simulink model "PMSM_SVC_RHF"  (R2019b)
settings: Solver=ode1  StartTime=0.0  StopTime=10  FixedStep=Tsim  RelTol=1e-3  EnableMultiTasking=on
PostLoadFcn:
  | , if any(exist('dsrtsu_mdlpostloadfcn', 'file') == [2, 3, 6]), try dsrtsu_mdlpostloadfcn('Execute', bdroot); catch fprintf('Error in PostLoadFcn (dsrtsu_mdlpostloadfcn) for model "%s":\n %s\n', bdroot, lasterr); end, end,
undefined symbols (not defined in the file or in its folder): bw_BPF, DiscIntNeverNeededParam, f_HF, Flux, fpwm, Fr, i_max, Jm, Ld, Lq, Ls, p, Rs, T_max, Tcur, Tsim, u_max, Udc, v_HF
libraries: powerlib x4, powerlib_meascontrol x4, simulink x1, powerlib_extras x1
settings Model: DSRTSU_INTERNAL_RTI_VER=490  DSRTSU_INTERNAL_RTI_TYPE=rti1202  SimulationMode=accelerator  Creator=XIL1XI  LastModifiedBy=LEI
settings SolverCC: AutoInsertRateTranBlk=on
settings DataIOCC: LimitDataPoints=on  ReturnWorkspaceOutputs=off
settings OptimizationCC: BlockReduction=off  OptimizeBlockIOStorage=off  BufferReuse=off  GlobalBufferReuse=off  ExpressionFolding=off  LocalBlockOutputs=off  LifeSpan=inf  OptimizeDataStoreBuffers=off  BusAssignmentInplaceUpdate=off
settings DebuggingCC: AllowSymbolicDim=off  SFUnexpectedBacktrackingDiag=warning  SFNoUnconditionalDefaultTransitionDiag=warning  SFExecutionAtInitializationDiag=none  ArithmeticOperatorsInVariantConditions=warning
settings HardwareCC: ProdBitPerPointer=32  ProdBitPerSizeT=32  ProdBitPerPtrDiffT=32  ProdLargestAtomicInteger=Integer  ProdEndianess=BigEndian  ProdWordSize=32  ProdHWDeviceType=Custom Processor->Custom
settings ModelReferenceCC: PropagateSignalLabelsOutOfModel=off
settings SFSimCC: SimUseLocalCustomCode=off  CustomCodeUndefinedFunction=UseInterfaceOnly
settings RTWCC: Description=dSPACE DS1202 Hardware Platform  SystemTargetFile=rti1202.tlc  MakeCommand=make_rti  TemplateMakefile=rti1202.tmf  RTWUseLocalCustomCode=off
settings CodeAppCC: StateflowObjectComments=on
settings STFCustomTargetCC: ModelReferenceCompliant=off  ParMdlRefBuildCompliant=on  MatFileLogging=on  SystemTargetFile=rti1202.tlc
settings GRTTargetCC: TargetLangStandard=C89/C90 (ANSI)  ModelReferenceCompliant=off  CompOptLevelCompliant=off  ConcurrentExecutionCompliant=off  CombineOutputUpdateFcns=off  CPPClassGenCompliant=off  UseToolchainInfoCompliant=off
settings ConfigComp: CovMetricSettings=dw  CovHtmlReporting=on  CovSaveCumulativeToWorkspaceVar=on  CovSaveSingleToWorkspaceVar=on  CovExternalEMLEnable=off
settings SimscapeCC: SimscapeNormalizeSystem=off

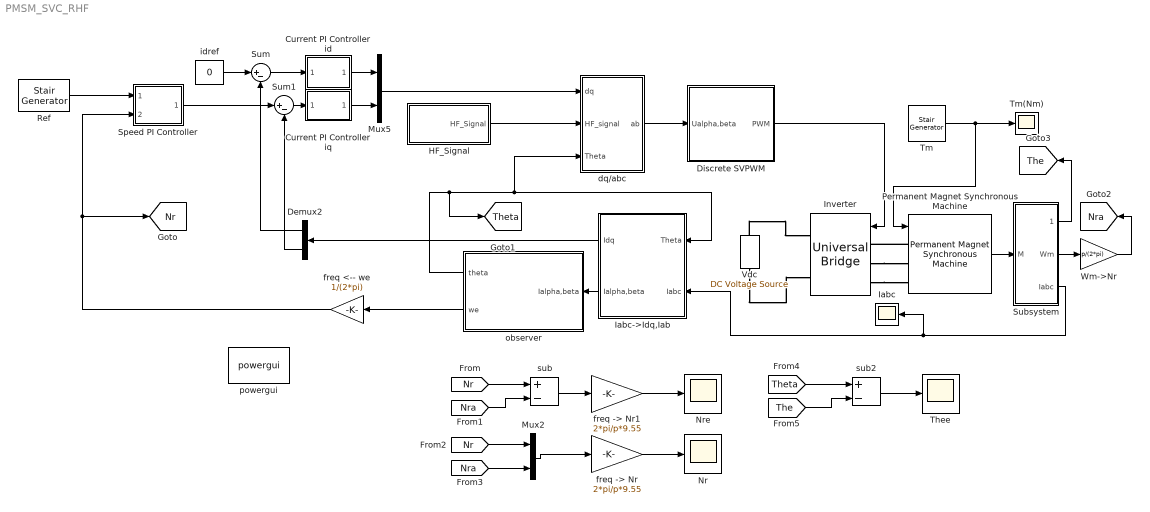
== system PMSM_SVC_RHF ==
  " Current PI Controller iq" : Subsystem  mask(Current PI Controller){Rs=Rs, Ls=Ld, fpwm=fpwm, Par_Limits=[u_max -u_max], T=Tcur, kp_gain=1, ti_gain=1}
      mask prompts: Rs "Stator resistance Rs (ohm):"; Ls "Stator inductance Ls (H):"; fpwm "PWM frequency fpwm (Hz):"; Par_Limits "Output limits Par_Limits (V): [ Upper   Lower ]"; T "Sample time T (s):"
      mask help:
      | Kp, Ti can be calculated automatically:
      |
      |     kp = Ls/2*fpwm;
      |     ti = Ls/Rs;
      |     ki = kp/ti;
      |
      | Kp_Gain, Ki_Gain are used to adjust the calculated kp and ki. Controller limit is the integrator saturation limit and the output limit.
      mask Display: disp('PI');
  Current PI Controller id : Subsystem  mask(Current PI Controller){Rs=Rs, Ls=Ld, fpwm=fpwm, Par_Limits=[u_max -u_max], T=Tcur, kp_gain=1, ti_gain=1}
      mask prompts: Rs "Stator resistance Rs (ohm):"; Ls "Stator inductance Ls (H):"; fpwm "PWM frequency fpwm (Hz):"; Par_Limits "Output limits Par_Limits (V): [ Upper   Lower ]"; T "Sample time T (s):"
      mask help:
      | Kp, Ti can be calculated automatically:
      |
      |     kp = Ls/2*fpwm;
      |     ti = Ls/Rs;
      |     ki = kp/ti;
      |
      | Kp_Gain, Ki_Gain are used to adjust the calculated kp and ki. Controller limit is the integrator saturation limit and the output limit.
      mask Display: disp('PI');
  Demux2 : Demux  Outputs=2
  Discrete SVPWM : Subsystem  mask(Seven - sects SVPWM generator){td=0, fpwm=fpwm, T=Tsim}
      mask prompts: td "Dead Time td (s):"; fpwm "PWM frequency fpwm (Hz):"; T "Sample time T (s):"
      mask help: This block implements a space vector PWM.
  HF_Signal : Subsystem
  Iabc : Scope
  Iabc->Idq,Iab : Subsystem  mask(Transformation abc to ab and dq){T=Tcur}
      mask prompts: T "Sample time T (s):"
  Inverter : powerlib/Power Electronics/Universal Bridge  Arms=3  SnubberResistance=1e5  SnubberCapacitance=inf  Device=IGBT / Diodes  Ron=1e-3  Lon=0  ForwardVoltages=[0,0]  ForwardVoltage=0  GTOparameters=[ 10e-6 , 20e-6 ]  IGBTparameters=[0,0]  Measurements=None  Measurements_2=None  converterType=Rectifier
      settings: SourceProductName=Simscape Electrical
  Mux2 : Mux  Inputs=2
  Mux5 : Mux  Inputs=2
  Nr : Scope
  Nre : Scope
  Permanent Magnet Synchronous Machine : powerlib/Machines/Permanent Magnet Synchronous Machine  NbPhases=3  FluxDistribution=Sinusoidal  RotorType=Salient-pole  MechanicalLoad=Torque Tm  PresetModel=No  ShowDetailedParameters=on  MeasurementBus=off  Resistance=Rs  Inductance=8.5e-3  dqInductances=[Ld,Lq]  La=Ls  MachineConstant=Flux linkage established by magnets (V.s)  Flux=Flux  VoltageCst=161.7909  TorqueCst=1.338  Flat=120  Mechanical=[Jm Fr p 0]  PolePairs=4  InitialConditions=[0,0, 0,0]  InitialConditions5ph=[0 0 0 0 0 0]  RefAngle=Aligned with phase A axis (original Park)  IterativeDiscreteModel=Trapezoidal non iterative  TsBlock=-1  TsPowergui=0
  Ref : powerlib_meascontrol/Pulse & Signal Generators/Stair Generator  t="[0  2  6 ]"  e=[0 10 20]  Ts=Tcur
      settings: SourceProductName=Simscape Electrical
  Speed PI Controller : Subsystem  mask(Speed PI Controller){kp=2.5, ti=2.5/10, Par_Limits=[T_max -T_max], T=Tcur}
      mask prompts: kp "proportional gain"; ti "integral time"; Par_Limits "Output limits: [ Upper   Lower ]"; T "Sample time T (s):"
      mask help:
      | Kp, Ti can be calculated automatically:
      |
      |     kp = Jm*(h+1)/(2*h*2*fpwm*kt)*kp_gain;
      |     ki = Jm*(h+1)/(2*h*2*fpwm*kt)/(2*1/fpwm)*ti_gain;
      |     ti = kp/ki;
      |
      |
      | Kp_Gain, Ki_Gain are used to adjust the calculated kp and ki. Controller limit is the integrator saturation limit and the output limit.
      mask init:
      | UpperLimit=Par_Limits(1);
      | LowerLimit=Par_Limits(2);
      | 
      | ki = kp/ti;
      mask Display: disp('PI')
  Subsystem : Subsystem
  Sum : Sum  Inputs=|+-
  Sum1 : Sum  Inputs=|+-
  Thee : Scope
  Tm : powerlib_meascontrol/Pulse & Signal Generators/Stair Generator  t="[0  4 ]"  e=[0 3 ]  Ts=0
      settings: SourceProductName=Simscape Electrical
  Tm(Nm) : Scope
  Vdc : powerlib/Electrical Sources/DC Voltage Source  Amplitude=Udc  Measurements=None
      settings: SourceProductName=Simscape Electrical
  Wm->Nr : Gain  Gain=p/(2*pi)
  dq/abc : Subsystem
  "freq -> Nr" : Gain  Gain=2*pi/p*9.55
  "freq -> Nr1" : Gain  Gain=2*pi/p*9.55
  freq <-- we : Gain  Gain=1/(2*pi)
  idref : Constant  Value=0
  observer : Subsystem
  powergui : powerlib/powergui  Priority=1  SimulationMode=Discrete  SampleTime=Tsim  frequency=60  Iterations=50  frequencyindice=0  Pbase=100e6  ErrMax=1e-4  UnitsV=kV  UnitsW=MW  buscounter=0  FunctionMessages=off  echomessages=off  EnableUseOfTLC=off  CurrentSourceSwitches=off  DisableSnubberDevices=off  DisableRonSwitches=off  DisableVfSwitches=off  DisplayEquations=off  AutomaticDiscreteSolvers=off  SolverType=Tustin/Backward Euler (TBE)  Interpol=off  ExternalGateDelay=off  methode=off  Ts=10  x0status=blocks  SPID=off  SwTol=0  HookPort=off  NonlinearTolerance=1e-4  nMaxIteration=100  ContinueOnMaxIteration=off  RestoreLinks=warning  ResistiveCurrentMeasurement=off  Frange=[0:2:500]  Ylog=off  Xlog=on  ShowGrid=off  save=off  variable=ZData  structure=0  ZoomFFT=off  StartTime=0.0  cycles=1  DisplayStyle=1  fundamental=60  FreqAxis=off  MaxFrequency=1000  frequencyindicesteady=1  RmsSteady=1  display=off
      settings: SourceProductName=Simscape Electrical
  sub : Sum  Inputs=+-
  sub2 : Sum  Inputs=+-
  tag scope: Nr=global, Nra=global, The=global, Theta=global
  wires:
  Current PI Controller id/1(U_Ref) -> Mux5/1
  " Current PI Controller iq"/1(U_Ref) -> Mux5/2
  observer/2(we) -> freq <-- we/1
  Mux2/1 -> "freq -> Nr"/1
  Mux5/1 -> dq/abc/1(dq)
  dq/abc/1(ab) -> Discrete SVPWM/1(Ualpha,beta)
  Iabc->Idq,Iab/1(Idq) -> Demux2/1
  Iabc->Idq,Iab/2(Ialpha,beta) -> observer/1(Ialpha,beta)
  Tm/1 -> Permanent Magnet Synchronous Machine/1, Tm(Nm)/1
  sub/1 -> "freq -> Nr1"/1
  Ref/1 -> Speed PI Controller/1(f_ref)
  Permanent Magnet Synchronous Machine/1 -> Subsystem/1(M)
  HF_Signal/1(HF_Signal) -> dq/abc/2(HF_signal)
  Discrete SVPWM/1(PWM) -> Inverter/1
  Subsystem/3(Iabc) -> Iabc/1, Iabc->Idq,Iab/2(Iabc)
  "freq -> Nr"/1 -> Nr/1
  "freq -> Nr1"/1 -> Nre/1
  Demux2/1 -> Sum/2
  Subsystem/2(Wm) -> Wm->Nr/1
  observer/1(theta) -> [Theta], Iabc->Idq,Iab/1(Theta), dq/abc/3(Theta)
  freq <-- we/1 -> [Nr], Speed PI Controller/2(f_fed)
  [Nr] -> sub/1
  Wm->Nr/1 -> [Nra]
  [Nra] -> sub/2
  [Nr] -> Mux2/1
  [Nra] -> Mux2/2
  Subsystem/1(Them) -> [The]
  [Theta] -> sub2/1
  [The] -> sub2/2
  sub2/1 -> Thee/1
  Sum/1 -> Current PI Controller id/1(I_Ref)
  Sum1/1 -> " Current PI Controller iq"/1(I_Ref)
  Speed PI Controller/1(Te_Ref) -> Sum1/1
  Demux2/2 -> Sum1/2
  idref/1 -> Sum/1
  connections:
  Inverter/LConn2 -- Permanent Magnet Synchronous Machine/LConn2
  Permanent Magnet Synchronous Machine/LConn1 -- Inverter/LConn1
  Inverter/LConn3 -- Permanent Magnet Synchronous Machine/LConn3
  Vdc/RConn1 -- Inverter/RConn1
  Vdc/LConn1 -- Inverter/RConn2

== system PMSM_SVC_RHF/ Current PI Controller iq ==
  I_Ref : Inport
  Discrete-Time Integrator1 : DiscreteIntegrator  IntegratorMethod=Integration: Trapezoidal  SampleTime=T  LimitOutput=on  UpperSaturationLimit=Par_Limits(1)  LowerSaturationLimit=Par_Limits(2)  ICPrevOutput=DiscIntNeverNeededParam  ICPrevScaledInput=DiscIntNeverNeededParam
  Output limit : Saturate  UpperLimit=Par_Limits(1)  LowerLimit=Par_Limits(2)
  Sum1 : Sum  Inputs=|++
  ki : Gain  Gain=(Ls/2*fpwm)/(Ls/Rs)*kp_gain/ti_gain
  kp : Gain  Gain=(Ls/2*fpwm)*kp_gain
  U_Ref : Outport  VectorParamsAs1DForOutWhenUnconnected=off
  wires:
  kp/1 -> Sum1/1
  I_Ref/1 -> ki/1, kp/1
  Sum1/1 -> Output limit/1
  Output limit/1 -> U_Ref/1
  Discrete-Time Integrator1/1 -> Sum1/2
  ki/1 -> Discrete-Time Integrator1/1

== system PMSM_SVC_RHF/Current PI Controller id ==
  I_Ref : Inport
  Discrete-Time Integrator1 : DiscreteIntegrator  IntegratorMethod=Integration: Trapezoidal  SampleTime=T  LimitOutput=on  UpperSaturationLimit=Par_Limits(1)  LowerSaturationLimit=Par_Limits(2)  ICPrevOutput=DiscIntNeverNeededParam  ICPrevScaledInput=DiscIntNeverNeededParam
  Output limit : Saturate  UpperLimit=Par_Limits(1)  LowerLimit=Par_Limits(2)
  Sum1 : Sum  Inputs=|++
  ki : Gain  Gain=(Ls/2*fpwm)/(Ls/Rs)*kp_gain/ti_gain
  kp : Gain  Gain=(Ls/2*fpwm)*kp_gain
  U_Ref : Outport  VectorParamsAs1DForOutWhenUnconnected=off
  wires:
  kp/1 -> Sum1/1
  I_Ref/1 -> ki/1, kp/1
  Sum1/1 -> Output limit/1
  Output limit/1 -> U_Ref/1
  Discrete-Time Integrator1/1 -> Sum1/2
  ki/1 -> Discrete-Time Integrator1/1

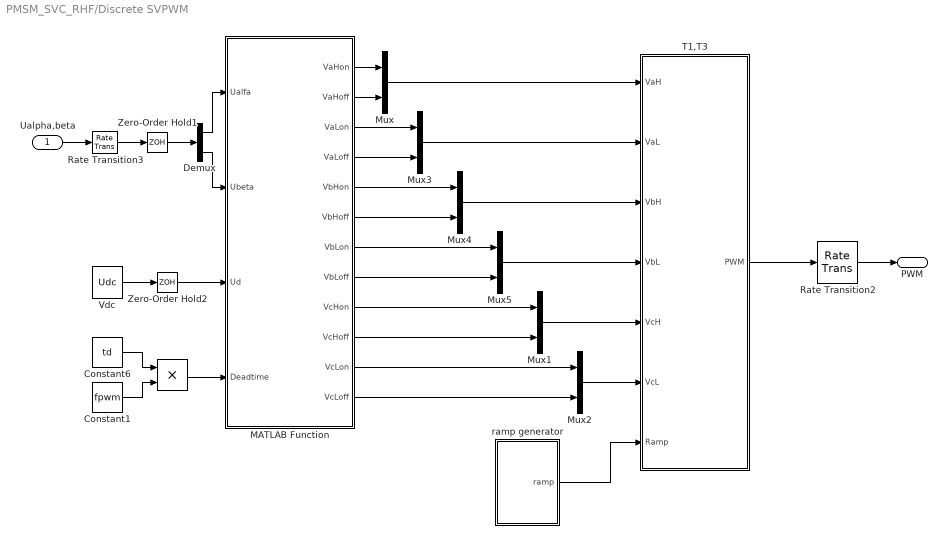
== system PMSM_SVC_RHF/Discrete SVPWM ==
  Ualpha,beta : Inport
  " " : Product  RndMeth=Zero
  Constant1 : Constant  Value=fpwm
  Constant6 : Constant  Value=td
  Demux : Demux  Outputs=2
  MATLAB Function : MATLAB Function  TreatAsAtomicUnit=on
  Mux{,1..5} (6 alike) : Mux  Inputs=2
  Rate Transition2 : RateTransition
  Rate Transition3 : RateTransition  OutPortSampleTime=Tsim
  T1,T3 : Subsystem
  "Vdc " : Constant  Value=Udc
  Zero-Order Hold1 : ZeroOrderHold  SampleTime=T
  Zero-Order Hold2 : ZeroOrderHold  SampleTime=T
  ramp generator : Subsystem
  PWM : Outport  VectorParamsAs1DForOutWhenUnconnected=off
  wires:
  Constant1/1 -> " "/2
  Demux/2 -> MATLAB Function/2(Ubeta)
  Demux/1 -> MATLAB Function/1(Ualfa)
  Zero-Order Hold1/1 -> Demux/1
  Zero-Order Hold2/1 -> MATLAB Function/3(Ud)
  Rate Transition2/1 -> PWM/1
  T1,T3/1(PWM) -> Rate Transition2/1
  ramp generator/1(ramp) -> T1,T3/7(Ramp)
  Mux2/1 -> T1,T3/6(VcL)
  MATLAB Function/12(VcLoff) -> Mux2/2
  MATLAB Function/11(VcLon) -> Mux2/1
  Mux1/1 -> T1,T3/5(VcH)
  MATLAB Function/10(VcHoff) -> Mux1/2
  MATLAB Function/9(VcHon) -> Mux1/1
  Mux5/1 -> T1,T3/4(VbL)
  MATLAB Function/8(VbLoff) -> Mux5/2
  MATLAB Function/7(VbLon) -> Mux5/1
  Mux4/1 -> T1,T3/3(VbH)
  MATLAB Function/6(VbHoff) -> Mux4/2
  MATLAB Function/5(VbHon) -> Mux4/1
  Mux3/1 -> T1,T3/2(VaL)
  MATLAB Function/4(VaLoff) -> Mux3/2
  MATLAB Function/3(VaLon) -> Mux3/1
  Mux/1 -> T1,T3/1(VaH)
  " "/1 -> MATLAB Function/4(Deadtime)
  Constant6/1 -> " "/1
  MATLAB Function/2(VaHoff) -> Mux/2
  MATLAB Function/1(VaHon) -> Mux/1
  "Vdc "/1 -> Zero-Order Hold2/1
  Ualpha,beta/1 -> Rate Transition3/1
  Rate Transition3/1 -> Zero-Order Hold1/1

== system PMSM_SVC_RHF/HF_Signal ==
  Cos Wave : Sin  Amplitude=v_HF  Frequency=2*pi*f_HF  Phase=pi/2  SampleTime=Tcur
  Gain1 : Gain  Gain=-1
  Mux : Mux  Inputs=2
  Rate Transition7 : RateTransition
  Sine : Sin  Amplitude=v_HF  Frequency=2*pi*f_HF  SampleTime=Tcur
  Zero-Order Hold6 : ZeroOrderHold  SampleTime=Tcur
  HF_Signal : Outport  VectorParamsAs1DForOutWhenUnconnected=off
  wires:
  Gain1/1 -> Mux/1
  Cos Wave/1 -> Mux/2
  Sine/1 -> Gain1/1
  Rate Transition7/1 -> Zero-Order Hold6/1
  Mux/1 -> Rate Transition7/1
  Zero-Order Hold6/1 -> HF_Signal/1

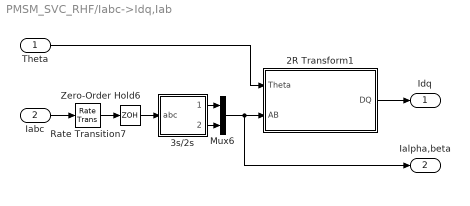
== system PMSM_SVC_RHF/Iabc->Idq,Iab ==
  Theta : Inport
  Iabc : Inport  Port=2
  2R Transform1 : Subsystem  mask(2S/2R Transform){}
      mask help:
      | -> D = Alpha *cos(Theta)+ Beta *sin(Theta)
      | -> Q = -Alpha *sin(Theta)+ Beta *cos(Theta)
      mask Display: fprintf('2S/2R', 17)
  3s/2s : Subsystem
  Mux6 : Mux  Inputs=2
  Rate Transition7 : RateTransition
  Zero-Order Hold6 : ZeroOrderHold  SampleTime=T
  Idq : Outport  VectorParamsAs1DForOutWhenUnconnected=off
  Ialpha,beta : Outport  Port=2  VectorParamsAs1DForOutWhenUnconnected=off
  wires:
  Iabc/1 -> Rate Transition7/1
  Zero-Order Hold6/1 -> 3s/2s/1(abc)
  3s/2s/1(alpha) -> Mux6/1
  3s/2s/2(beta) -> Mux6/2
  2R Transform1/1(DQ) -> Idq/1
  Mux6/1 -> Ialpha,beta/1, 2R Transform1/2(AB)
  Theta/1 -> 2R Transform1/1(Theta)
  Rate Transition7/1 -> Zero-Order Hold6/1

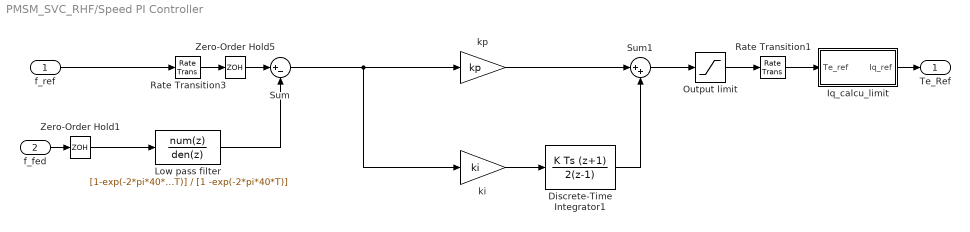
== system PMSM_SVC_RHF/Speed PI Controller ==
  f_ref : Inport
  f_fed : Inport  Port=2
  Discrete-Time Integrator1 : DiscreteIntegrator  IntegratorMethod=Integration: Trapezoidal  SampleTime=T  LimitOutput=on  UpperSaturationLimit=UpperLimit  LowerSaturationLimit=LowerLimit  ICPrevOutput=DiscIntNeverNeededParam  ICPrevScaledInput=DiscIntNeverNeededParam
  Iq_calcu_limit : Subsystem
  Low pass filter : DiscreteTransferFcn  Numerator=[1-exp(-2*pi*40*T)]  Denominator=[1 -exp(-2*pi*40*T)]  SampleTime=T
  Output limit : Saturate  UpperLimit=UpperLimit  LowerLimit=LowerLimit
  Rate Transition1 : RateTransition
  Rate Transition3 : RateTransition
  Sum : Sum  Inputs=|+-
  Sum1 : Sum  Inputs=|++
  Zero-Order Hold1 : ZeroOrderHold  SampleTime=T
  Zero-Order Hold5 : ZeroOrderHold  SampleTime=T
  ki : Gain  Gain=ki
  kp : Gain  Gain=kp
  Te_Ref : Outport  VectorParamsAs1DForOutWhenUnconnected=off
  wires:
  ki/1 -> Discrete-Time Integrator1/1
  Discrete-Time Integrator1/1 -> Sum1/2
  Sum1/1 -> Output limit/1
  Sum/1 -> kp/1, ki/1
  kp/1 -> Sum1/1
  f_ref/1 -> Rate Transition3/1
  Rate Transition3/1 -> Zero-Order Hold5/1
  Zero-Order Hold5/1 -> Sum/1
  f_fed/1 -> Zero-Order Hold1/1
  Zero-Order Hold1/1 -> Low pass filter/1
  Output limit/1 -> Rate Transition1/1
  Rate Transition1/1 -> Iq_calcu_limit/1(Te_ref)
  Low pass filter/1 -> Sum/2
  Iq_calcu_limit/1(Iq_ref) -> Te_Ref/1

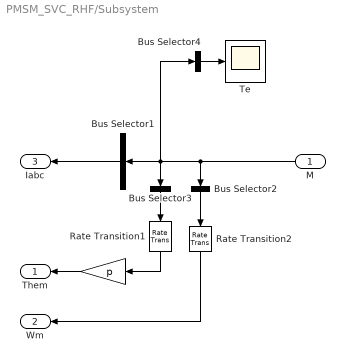
== system PMSM_SVC_RHF/Subsystem ==
  M : Inport
  " " : Gain  Gain=p  SaturateOnIntegerOverflow=on  OutDataTypeStr=Inherit: Same as input  ParamDataTypeStr=Inherit: Same as input
  Bus Selector1 : BusSelector  OutputSignals=Stator current is_a (A),Stator current is_b (A),Stator current is_c (A)  OutputAsBus=on
  Bus Selector2 : BusSelector  OutputSignals=Rotor speed wm (rad/s)  OutputAsBus=on
  Bus Selector3 : BusSelector  OutputSignals=Rotor angle thetam (rad)  OutputAsBus=on
  Bus Selector4 : BusSelector  OutputSignals=Electromagnetic torque Te (N*m)  OutputAsBus=on
  Rate Transition1 : RateTransition  OutPortSampleTime=Tcur
  Rate Transition2 : RateTransition  OutPortSampleTime=Tcur
  Te : Scope
  Them : Outport  VectorParamsAs1DForOutWhenUnconnected=off
  Wm : Outport  Port=2  VectorParamsAs1DForOutWhenUnconnected=off
  Iabc : Outport  Port=3  VectorParamsAs1DForOutWhenUnconnected=off
  wires:
  M/1 -> Bus Selector4/1, Bus Selector3/1, Bus Selector1/1, Bus Selector2/1
  Bus Selector3/1 -> Rate Transition1/1
  Bus Selector1/1 -> Iabc/1
  Bus Selector2/1 -> Rate Transition2/1
  Rate Transition2/1 -> Wm/1
  Rate Transition1/1 -> " "/1
  " "/1 -> Them/1
  Bus Selector4/1 -> Te/1

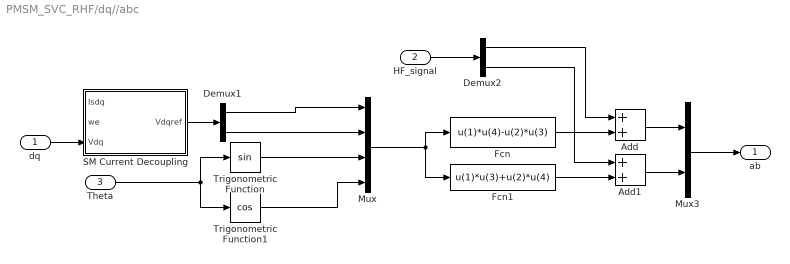
== system PMSM_SVC_RHF/dq//abc ==
  dq : Inport
  HF_signal : Inport  Port=2
  Theta : Inport  Port=3
  " SM Current Decoupling" : Subsystem  mask(SM Feedforward Decoupling){Rs=Rs, Ls=Ls, Flux=Flux, Par_Limits=[u_max -u_max], T=Tcur}
      mask prompts: Rs "The stator resistance /ohm:"; Ls "The stator inductance /H:"; Flux "The flux linkage established by magnets /Wb"; Par_Limits "Output voltage limit (V): [ Upper  Lower ]"; T "Sample time T (s):"
      mask help:
      | This module is a current decoupling scheme:
      | -> Vd_Ref = Vd + (d-axis decoupling part)
      | -> Vq_Ref = Vq + (q-axis decoupling part)
      | The total output is limited according to parameter setting.
      mask init:
      | UpperLimit=Par_Limits(1);
      | LowerLimit=Par_Limits(2);
  Add : Sum
  Add1 : Sum
  Demux1 : Demux  Outputs=2
  Demux2 : Demux  Outputs=2
  Fcn : Fcn  Expr=u(1)*u(4)-u(2)*u(3)
  Fcn1 : Fcn  Expr=u(1)*u(3)+u(2)*u(4)
  Mux : Mux
  Mux3 : Mux  Inputs=2
  Trigonometric Function : Trigonometry
  Trigonometric Function1 : Trigonometry  Operator=cos
  ab : Outport  VectorParamsAs1DForOutWhenUnconnected=off
  wires:
  Theta/1 -> Trigonometric Function1/1, Trigonometric Function/1
  Trigonometric Function1/1 -> Mux/4
  Trigonometric Function/1 -> Mux/3
  Demux1/2 -> Mux/2
  Demux1/1 -> Mux/1
  Mux/1 -> Fcn1/1, Fcn/1
  Mux3/1 -> ab/1
  Fcn/1 -> Add/2
  Add/1 -> Mux3/1
  Fcn1/1 -> Add1/2
  Add1/1 -> Mux3/2
  HF_signal/1 -> Demux2/1
  Demux2/1 -> Add/1
  Demux2/2 -> Add1/1
  dq/1 -> " SM Current Decoupling"/3(Vdq)
  " SM Current Decoupling"/1(Vdqref) -> Demux1/1

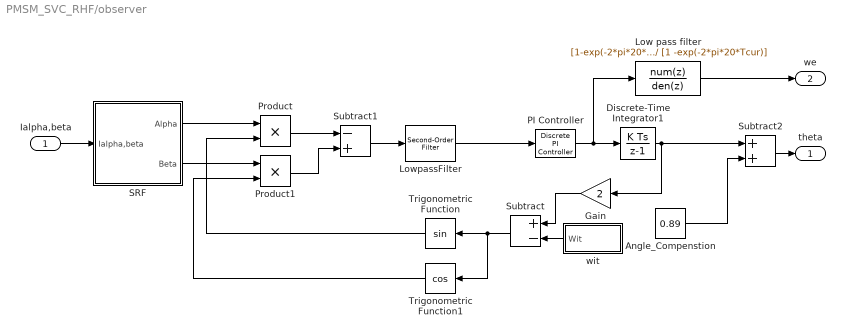
== system PMSM_SVC_RHF/observer ==
  Ialpha,beta : Inport
  Angle_Compenstion : Constant  Value=0.89
  Discrete-Time Integrator1 : DiscreteIntegrator  InitialCondition=0.09  SampleTime=-1  ICPrevOutput=DiscIntNeverNeededParam  ICPrevScaledInput=DiscIntNeverNeededParam
  Gain : Gain  Gain=2
  Low pass filter : DiscreteTransferFcn  Numerator=[1-exp(-2*pi*20*Tcur)]  Denominator=[1 -exp(-2*pi*20*Tcur)]  SampleTime=Tcur
  LowpassFilter : powerlib_meascontrol/Filters/Second-Order Filter  FilterType=Lowpass  Fo=500  Zeta=0.707  Ts=Tcur  Initialize=off  Vac_Init="[0,  0,  60]"  Vdc_Init=0  PlotResponse=off  FreqRange=[0, 500, 1]
      settings: SourceProductName=Simscape Electrical  SourceProductBaseCode=PS
  PI Controller : powerlib_extras/Discrete  Control Blocks/Discrete PI Controller  Kp=25  Ki=600  Par_Limits=[100*2*pi -100*2*pi]  Init=0  Ts=Tcur
      settings: SourceProductName=Simscape Electrical
  Product : Product
  Product1 : Product
  SRF : Subsystem
  Subtract : Sum  Inputs=+-
  Subtract1 : Sum  Inputs=-+
  Subtract2 : Sum
  Trigonometric Function : Trigonometry
  Trigonometric Function1 : Trigonometry  Operator=cos
  wit : Subsystem
  theta : Outport  VectorParamsAs1DForOutWhenUnconnected=off
  we : Outport  Port=2  VectorParamsAs1DForOutWhenUnconnected=off
  wires:
  Subtract1/1 -> LowpassFilter/1
  LowpassFilter/1 -> PI Controller/1
  PI Controller/1 -> Low pass filter/1, Discrete-Time Integrator1/1
  Discrete-Time Integrator1/1 -> Subtract2/1, Gain/1
  Low pass filter/1 -> we/1
  Ialpha,beta/1 -> SRF/1(Ialpha,beta)
  SRF/1(Alpha) -> Product/1
  wit/1(Wit) -> Subtract/2
  Gain/1 -> Subtract/1
  Subtract/1 -> Trigonometric Function1/1, Trigonometric Function/1
  Trigonometric Function/1 -> Product/2
  SRF/2(Beta) -> Product1/1
  Trigonometric Function1/1 -> Product1/2
  Product1/1 -> Subtract1/2
  Product/1 -> Subtract1/1
  Subtract2/1 -> theta/1
  Angle_Compenstion/1 -> Subtract2/2

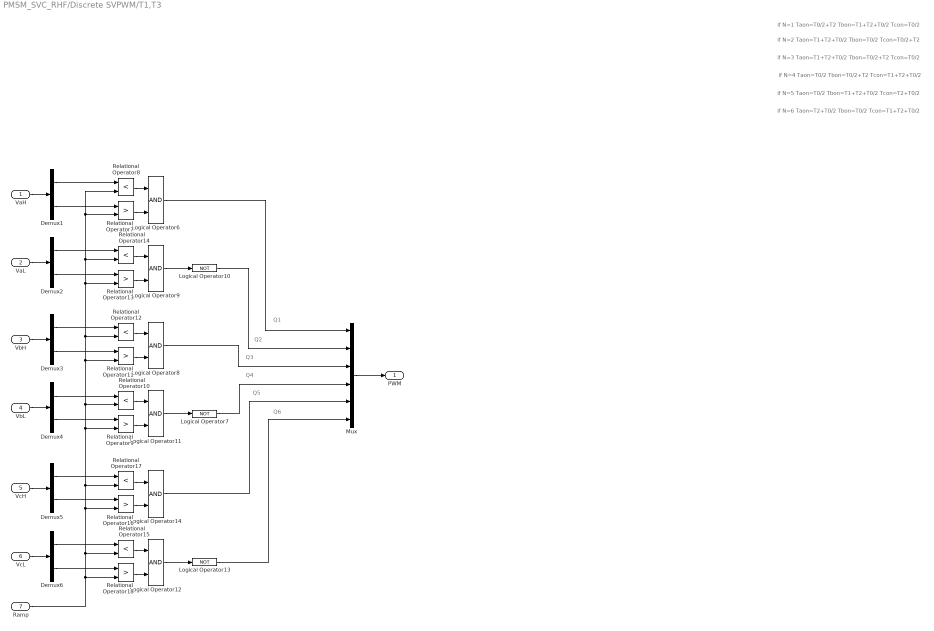
== system PMSM_SVC_RHF/Discrete SVPWM/T1,T3 ==
  note: if N=6 Taon=T2+T0/2 Tbon=T0/2 Tcon=T1+T2+T0/2
  note: if N=5 Taon=T0/2 Tbon=T1+T2+T0/2 Tcon=T2+T0/2
  note: if N=4 Taon=T0/2 Tbon=T0/2+T2 Tcon=T1+T2+T0/2
  note: if N=3 Taon=T1+T2+T0/2 Tbon=T0/2+T2 Tcon=T0/2
  note: if N=2 Taon=T1+T2+T0/2 Tbon=T0/2 Tcon=T0/2+T2
  note: if N=1 Taon=T0/2+T2 Tbon=T1+T2+T0/2 Tcon=T0/2
  note: Q1
  note: Q2
  note: Q3
  note: Q4
  note: Q5
  note: Q6
  VaH : Inport
  VaL : Inport  Port=2
  VbH : Inport  Port=3
  VbL : Inport  Port=4
  VcH : Inport  Port=5
  VcL : Inport  Port=6
  Ramp : Inport  Port=7
  Demux{1..6} (6 alike) : Demux  Outputs=2
  Logical Operator10 : Logic  Operator=NOT
  Logical Operator{6,8..9,11..12,14} (6 alike) : Logic
  Logical Operator13 : Logic  Operator=NOT
  Logical Operator7 : Logic  Operator=NOT
  Mux : Mux  Inputs=6
  Relational Operator{8,10,12,14..15,17} (6 alike) : RelationalOperator  Operator=<  RndMeth=Nearest  InputSameDT=on
  Relational Operator{7,9,11,13,16,18} (6 alike) : RelationalOperator  Operator=>  RndMeth=Nearest  InputSameDT=on
  PWM : Outport  VectorParamsAs1DForOutWhenUnconnected=off
  wires:
  Logical Operator13/1 -> Mux/6
  Logical Operator14/1 -> Mux/5
  Logical Operator7/1 -> Mux/4
  Logical Operator8/1 -> Mux/3
  Logical Operator10/1 -> Mux/2
  Logical Operator6/1 -> Mux/1
  Ramp/1 -> Relational Operator12/2, Relational Operator8/2, Relational Operator7/2, Relational Operator14/2, Relational Operator13/2, Relational Operator11/2, Relational Operator10/2, Relational Operator9/2, Relational Operator17/2, Relational Operator16/2, Relational Operator15/2, Relational Operator18/2
  Logical Operator12/1 -> Logical Operator13/1
  Demux6/1 -> Relational Operator15/1
  VcL/1 -> Demux6/1
  Demux6/2 -> Relational Operator18/1
  Relational Operator18/1 -> Logical Operator12/2
  Relational Operator15/1 -> Logical Operator12/1
  VcH/1 -> Demux5/1
  Demux5/2 -> Relational Operator16/1
  Relational Operator16/1 -> Logical Operator14/2
  Demux5/1 -> Relational Operator17/1
  Relational Operator17/1 -> Logical Operator14/1
  Logical Operator11/1 -> Logical Operator7/1
  Demux4/1 -> Relational Operator10/1
  VbL/1 -> Demux4/1
  Demux4/2 -> Relational Operator9/1
  Relational Operator9/1 -> Logical Operator11/2
  Relational Operator10/1 -> Logical Operator11/1
  VbH/1 -> Demux3/1
  Demux3/2 -> Relational Operator11/1
  Relational Operator11/1 -> Logical Operator8/2
  Demux3/1 -> Relational Operator12/1
  Relational Operator12/1 -> Logical Operator8/1
  Logical Operator9/1 -> Logical Operator10/1
  Demux2/1 -> Relational Operator14/1
  VaL/1 -> Demux2/1
  Demux2/2 -> Relational Operator13/1
  Relational Operator13/1 -> Logical Operator9/2
  Relational Operator14/1 -> Logical Operator9/1
  VaH/1 -> Demux1/1
  Demux1/2 -> Relational Operator7/1
  Relational Operator7/1 -> Logical Operator6/2
  Demux1/1 -> Relational Operator8/1
  Relational Operator8/1 -> Logical Operator6/1
  Mux/1 -> PWM/1

== system PMSM_SVC_RHF/Discrete SVPWM/ramp generator ==
  Constant1 : Constant  Value=fpwm
  Constant3 : Constant  Value=1-1.5*T*fpwm
  Discrete-Time Integrator1 : DiscreteIntegrator  ExternalReset=rising  SampleTime=T  ICPrevOutput=DiscIntNeverNeededParam  ICPrevScaledInput=DiscIntNeverNeededParam
  Relational Operator1 : RelationalOperator  RndMeth=Nearest  InputSameDT=on
  Unit Delay1 : UnitDelay  SampleTime=T  HasFrameUpgradeWarning=on
  ramp : Outport  VectorParamsAs1DForOutWhenUnconnected=off
  wires:
  Discrete-Time Integrator1/1 -> Relational Operator1/1, ramp/1
  Unit Delay1/1 -> Discrete-Time Integrator1/2
  Relational Operator1/1 -> Unit Delay1/1
  Constant3/1 -> Relational Operator1/2
  Constant1/1 -> Discrete-Time Integrator1/1

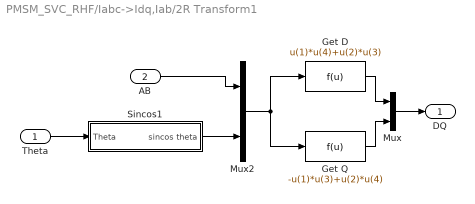
== system PMSM_SVC_RHF/Iabc->Idq,Iab/2R Transform1 ==
  Theta : Inport
  AB : Inport  Port=2
  Get D : Fcn  Expr=u(1)*u(4)+u(2)*u(3)
  Get Q : Fcn  Expr=-u(1)*u(3)+u(2)*u(4)
  Mux : Mux  Inputs=2
  Mux2 : Mux  Inputs=2
  Sincos1 : Subsystem  mask(2S/2R Transform){}
      mask help:
      | -> D = Alpha *cos(Theta)+ Beta *sin(Theta)
      | -> Q = -Alpha *sin(Theta)+ Beta *cos(Theta)
  DQ : Outport  VectorParamsAs1DForOutWhenUnconnected=off
  wires:
  Mux/1 -> DQ/1
  Get Q/1 -> Mux/2
  Get D/1 -> Mux/1
  Mux2/1 -> Get D/1, Get Q/1
  AB/1 -> Mux2/1
  Theta/1 -> Sincos1/1(Theta)
  Sincos1/1(sincos theta) -> Mux2/2

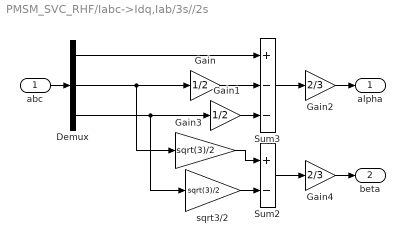
== system PMSM_SVC_RHF/Iabc->Idq,Iab/3s//2s ==
  abc : Inport
  Demux : Demux  Outputs=3
  Gain : Gain  Gain=1/2  SaturateOnIntegerOverflow=on  OutDataTypeStr=Inherit: Same as input  ParamDataTypeStr=Inherit: Same as input
  Gain1 : Gain  Gain=1/2  SaturateOnIntegerOverflow=on  OutDataTypeStr=Inherit: Same as input  ParamDataTypeStr=Inherit: Same as input
  Gain2 : Gain  Gain=2/3  SaturateOnIntegerOverflow=on  OutDataTypeStr=Inherit: Same as input  ParamDataTypeStr=Inherit: Same as input
  Gain3 : Gain  Gain=sqrt(3)/2  SaturateOnIntegerOverflow=on  OutDataTypeStr=Inherit: Same as input  ParamDataTypeStr=Inherit: Same as input
  Gain4 : Gain  Gain=2/3  SaturateOnIntegerOverflow=on  OutDataTypeStr=Inherit: Same as input  ParamDataTypeStr=Inherit: Same as input
  Sum2 : Sum  Inputs=+-  SaturateOnIntegerOverflow=on  InputSameDT=on  OutDataTypeStr=Inherit: Same as first input
  Sum3 : Sum  Inputs=+--  SaturateOnIntegerOverflow=on  InputSameDT=on  OutDataTypeStr=Inherit: Same as first input
  sqrt3/2 : Gain  Gain=sqrt(3)/2  SaturateOnIntegerOverflow=on  OutDataTypeStr=Inherit: Same as input  ParamDataTypeStr=Inherit: Same as input
  alpha : Outport  VectorParamsAs1DForOutWhenUnconnected=off
  beta : Outport  Port=2  VectorParamsAs1DForOutWhenUnconnected=off
  wires:
  Sum2/1 -> Gain4/1
  Gain2/1 -> alpha/1
  abc/1 -> Demux/1
  Demux/1 -> Sum3/1
  Demux/2 -> Gain/1, Gain3/1
  Gain1/1 -> Sum3/3
  Gain/1 -> Sum3/2
  Demux/3 -> Gain1/1, sqrt3/2/1
  Gain3/1 -> Sum2/1
  sqrt3/2/1 -> Sum2/2
  Gain4/1 -> beta/1
  Sum3/1 -> Gain2/1

== system PMSM_SVC_RHF/Speed PI Controller/Iq_calcu_limit ==
  Te_ref : Inport
  Fcn : Fcn  Expr=(2/3)*u/p/Flux
  Output limit1 : Saturate  UpperLimit=i_max  LowerLimit=-i_max
  Zero-Order Hold3 : ZeroOrderHold  SampleTime=Tcur
  Iq_ref : Outport  InitialOutput=0  VectorParamsAs1DForOutWhenUnconnected=off
  wires:
  Te_ref/1 -> Zero-Order Hold3/1
  Zero-Order Hold3/1 -> Fcn/1
  Fcn/1 -> Output limit1/1
  Output limit1/1 -> Iq_ref/1

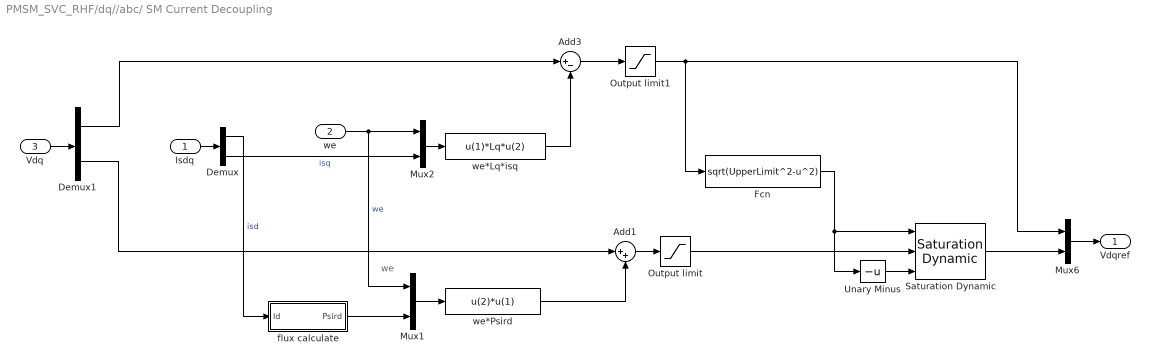
== system PMSM_SVC_RHF/dq//abc/ SM Current Decoupling ==
  note: we
  Isdq : Inport
  we : Inport  Port=2
  Vdq : Inport  Port=3
  Add1 : Sum  Inputs=|++  SampleTime=T
  Add3 : Sum  Inputs=|+-  SampleTime=T
  Demux : Demux  Outputs=2
  Demux1 : Demux  Outputs=2
  Fcn : Fcn  Expr=sqrt(UpperLimit^2-u^2)
  Mux1 : Mux  Inputs=2
  Mux2 : Mux  Inputs=2
  Mux6 : Mux  Inputs=2
  Output limit : Saturate  UpperLimit=UpperLimit  LowerLimit=LowerLimit
  Output limit1 : Saturate  UpperLimit=UpperLimit  LowerLimit=LowerLimit
  Saturation Dynamic : simulink/Discontinuities/Saturation Dynamic  OutMin=[]  OutMax=[]  OutDataTypeStr=Inherit: Same as second input  OutDataType=fixdt(1, 16)  OutScaling=2^-10  DoSatur=off
  Unary Minus : UnaryMinus
  flux calculate : Subsystem
  we*Lq*isq : Fcn  Expr=u(1)*Lq*u(2)  SampleTime=T
  we*Psird : Fcn  Expr=u(2)*u(1)  SampleTime=T
  Vdqref : Outport  VectorParamsAs1DForOutWhenUnconnected=off
  wires:
  flux calculate/1(Psird) -> Mux1/2
  Demux1/2 -> Add1/1
  Add3/1 -> Output limit1/1
  we*Lq*isq/1 -> Add3/2
  Demux1/1 -> Add3/1
  Output limit1/1 -> Fcn/1, Mux6/1
  Vdq/1 -> Demux1/1
  Mux1/1 -> we*Psird/1
  we/1 -> Mux2/1, Mux1/1  "we"
  Mux2/1 -> we*Lq*isq/1
  Add1/1 -> Output limit/1
  Demux/2 -> Mux2/2  "isq"
  Demux/1 -> flux calculate/1(Id)  "isd"
  Fcn/1 -> Unary Minus/1, Saturation Dynamic/1
  Unary Minus/1 -> Saturation Dynamic/3
  Output limit/1 -> Saturation Dynamic/2
  we*Psird/1 -> Add1/2
  Isdq/1 -> Demux/1
  Mux6/1 -> Vdqref/1
  Saturation Dynamic/1 -> Mux6/2

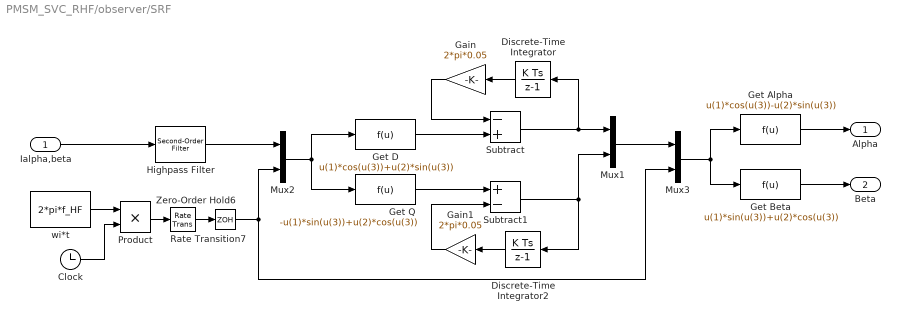
== system PMSM_SVC_RHF/observer/SRF ==
  Ialpha,beta : Inport
  Clock : Clock
  Discrete-Time Integrator : DiscreteIntegrator  SampleTime=Tcur  ICPrevOutput=DiscIntNeverNeededParam  ICPrevScaledInput=DiscIntNeverNeededParam
  Discrete-Time Integrator2 : DiscreteIntegrator  SampleTime=Tcur  ICPrevOutput=DiscIntNeverNeededParam  ICPrevScaledInput=DiscIntNeverNeededParam
  Gain : Gain  Gain=2*pi*0.05
  Gain1 : Gain  Gain=2*pi*0.05
  Get Alpha : Fcn  Expr=u(1)*cos(u(3))-u(2)*sin(u(3))
  Get Beta : Fcn  Expr=u(1)*sin(u(3))+u(2)*cos(u(3))
  Get D : Fcn  Expr=u(1)*cos(u(3))+u(2)*sin(u(3))
  Get Q : Fcn  Expr=-u(1)*sin(u(3))+u(2)*cos(u(3))
  Highpass Filter : powerlib_meascontrol/Filters/Second-Order Filter  FilterType=Highpass  Fo=f_HF - bw_BPF/2  Zeta=0.3  Ts=Tcur  Initialize=off  Vac_Init="[0,  0,  60]"  Vdc_Init=0  PlotResponse=off  FreqRange=[0, 10000, 1]
      settings: SourceProductName=Simscape Electrical  SourceProductBaseCode=PS
  Mux1 : Mux  Inputs=2
  Mux2 : Mux  Inputs=2
  Mux3 : Mux  Inputs=2
  Product : Product
  Rate Transition7 : RateTransition
  Subtract : Sum  Inputs=-+
  Subtract1 : Sum  Inputs=+-
  Zero-Order Hold6 : ZeroOrderHold  SampleTime=Tcur
  wi*t : Constant  Value=2*pi*f_HF
  Alpha : Outport  VectorParamsAs1DForOutWhenUnconnected=off
  Beta : Outport  Port=2  VectorParamsAs1DForOutWhenUnconnected=off
  wires:
  Subtract/1 -> Mux1/1, Discrete-Time Integrator/1
  Mux3/1 -> Get Alpha/1, Get Beta/1
  Mux1/1 -> Mux3/1
  Get Q/1 -> Subtract1/1
  Mux2/1 -> Get D/1, Get Q/1
  Clock/1 -> Product/2
  Discrete-Time Integrator2/1 -> Gain1/1
  wi*t/1 -> Product/1
  Discrete-Time Integrator/1 -> Gain/1
  Subtract1/1 -> Mux1/2, Discrete-Time Integrator2/1
  Get D/1 -> Subtract/2
  Gain1/1 -> Subtract1/2
  Get Alpha/1 -> Alpha/1
  Gain/1 -> Subtract/1
  Get Beta/1 -> Beta/1
  Rate Transition7/1 -> Zero-Order Hold6/1
  Product/1 -> Rate Transition7/1
  Zero-Order Hold6/1 -> Mux3/2, Mux2/2
  Ialpha,beta/1 -> Highpass Filter/1
  Highpass Filter/1 -> Mux2/1

== system PMSM_SVC_RHF/observer/wit ==
  Clock : Clock
  Product1 : Product
  Rate Transition7 : RateTransition
  Zero-Order Hold6 : ZeroOrderHold  SampleTime=Tcur
  wi*t : Constant  Value=2*pi*f_HF
  Wit : Outport  VectorParamsAs1DForOutWhenUnconnected=off
  wires:
  Clock/1 -> Product1/2
  wi*t/1 -> Product1/1
  Rate Transition7/1 -> Zero-Order Hold6/1
  Product1/1 -> Rate Transition7/1
  Zero-Order Hold6/1 -> Wit/1

== system PMSM_SVC_RHF/Iabc->Idq,Iab/2R Transform1/Sincos1 ==
  Theta : Inport
  Mux2 : Mux  Inputs=2
  Trigonometric Function : Trigonometry
  Trigonometric Function1 : Trigonometry  Operator=cos
  sincos theta : Outport  VectorParamsAs1DForOutWhenUnconnected=off
  wires:
  Mux2/1 -> sincos theta/1
  Theta/1 -> Trigonometric Function/1, Trigonometric Function1/1
  Trigonometric Function/1 -> Mux2/1
  Trigonometric Function1/1 -> Mux2/2

== system PMSM_SVC_RHF/dq//abc/ SM Current Decoupling/flux calculate ==
  Id : Inport
  Add2 : Sum  SampleTime=T
  Flux : Constant  Value=Flux
  Ld*id : Fcn  Expr=Ld*u(1)  SampleTime=T
  Scope5 : Scope
  Psird : Outport  VectorParamsAs1DForOutWhenUnconnected=off
  wires:
  Flux/1 -> Add2/2
  Add2/1 -> Psird/1, Scope5/1
  Ld*id/1 -> Add2/1
  Id/1 -> Ld*id/1

== matlab function PMSM_SVC_RHF/Discrete SVPWM/MATLAB Function ==
  data: Ualfa input; VaHon output; Ubeta input; Ud input; VaHoff output; VaLon output; VaLoff output; VbHon output; VbHoff output; VbLon output; VbLoff output; VcHon output; VcHoff output; Deadtime input; VcLon output; VcLoff output
function [VaHon,VaHoff,VaLon,VaLoff,VbHon,VbHoff,VbLon,VbLoff,VcHon,VcHoff,VcLon,VcLoff] = fcn(Ualfa,Ubeta,Ud,Deadtime)
%#codegen
X=1.732*Ubeta/Ud;
Y=(0.866*Ubeta+1.5*Ualfa)/Ud;
Z=(0.866*Ubeta-1.5*Ualfa)/Ud;
angle=atan2d(Ubeta,Ualfa);
if (angle>0)&&(angle<=60)   %N=3
   N=3;
   T1=-Z;
   T2=X;
else if (angle>60)&&(angle<=120)   %N=1
        N=1;
        T1=Z;
        T2=Y;
    else if(angle>120)&&(angle<=180)  %N=5
            N=5;
            T1=X;
            T2=-Y;
        else if(angle>-180)&&(angle<=-120)  %N=4
                N=4;
                T1=-X;
                T2=Z;
            else if(angle>-120)&&(angle<=-60)  %N=6
                    N=6;
                    T1=-Y;
                    T2=-Z;
                else  %N=2
                    N=2;
                    T1=Y;
                    T2=-X;
                end
            end
        end
    end
end

T=T1+T2;

if T>1
    T1=T1/T;
    T2=T2/T;
end

T0=1-T1-T2;

if N==3
    Taon=T1+T2+T0/2;
    Tbon=T0/2+T2;
    Tcon=T0/2;
else if N==1
         Taon=T0/2+T2;
         Tbon=T1+T2+T0/2;
         Tcon=T0/2;
     else if N==5
          Taon=T0/2;
          Tbon=T1+T2+T0/2;
          Tcon=T2+T0/2;
          else if N==4
               Taon=T0/2;
               Tbon=T0/2+T2;
               Tcon=T1+T2+T0/2;
               else if N==6
                    Taon=T2+T0/2;
                    Tbon=T0/2;
                    Tcon=T1+T2+T0/2;
                   else 
                        Taon=T1+T2+T0/2;
                        Tbon=T0/2;
                        Tcon=T0/2+T2;
                   end
               end
          end
    end
end

VaHon=(1-Taon)/2;
VaHoff=(1+Taon)/2;
if (VaHoff+Deadtime)>1  
    VaLon=0;
    VaLoff=1;
else if VaHoff==0.5
        VaLon=0.5;
        VaLoff=0.5;
    else
        VaLon=VaHon-Deadtime;
        VaLoff=VaHoff+Deadtime;
    end
end

VbHon=(1-Tbon)/2;
VbHoff=(1+Tbon)/2;

if (VbHoff+Deadtime)>1
    VbLon=0;
    VbLoff=1;
else if VbHoff==0.5
        VbLon=0.5;
        VbLoff=0.5;
    else
        VbLon=VbHon-Deadtime;
        VbLoff=VbHoff+Deadtime;
    end
end

VcHon=(1-Tcon)/2;
VcHoff=(1+Tcon)/2;

if (VcHoff+Deadtime)>1
    VcLon=0;
    VcLoff=1;
    else if VcHoff==0.5
            VcLon=0.5;
            VcLoff=0.5;
        else
            VcLon=VcHon-Deadtime;
            VcLoff=VcHoff+Deadtime;
        end
end
